simulink model "sun_vector_test_vallado"  (R2016b)
settings: Solver=VariableStepAuto  StartTime=0.0  StopTime=1  RelTol=1e-3
values from neighbouring files (symbols this model uses):
  JD_cent = (JD - J2000)/36525    (= -0.0487748117728)    [sun_vector_test_init.m]
  r_eci = [ 0; -4464.696; -5102.509 ] * 1e3    [sun_vector_test_init.m]
undefined symbols (not defined in the file or in its folder): sun_vector_lib
settings Model: Creator=taylorreynolds  LastModifiedBy=taylorreynolds

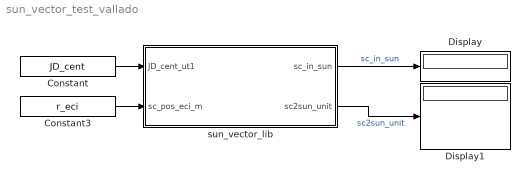
== system sun_vector_test_vallado ==
  Constant : Constant  Value=JD_cent
  Constant3 : Constant  Value=r_eci
  Display : Display
  Display1 : Display
  sun_vector_lib : Subsystem  AncestorBlock=sun_vector_lib/sun_vector_lib
  wires:
  Constant/1 -> sun_vector_lib/1(JD_cent_ut1)
  sun_vector_lib/1(sc_in_sun) -> Display/1  "sc_in_sun"
  sun_vector_lib/2(sc2sun_unit) -> Display1/1  "sc2sun_unit"
  Constant3/1 -> sun_vector_lib/2(sc_pos_eci_m)

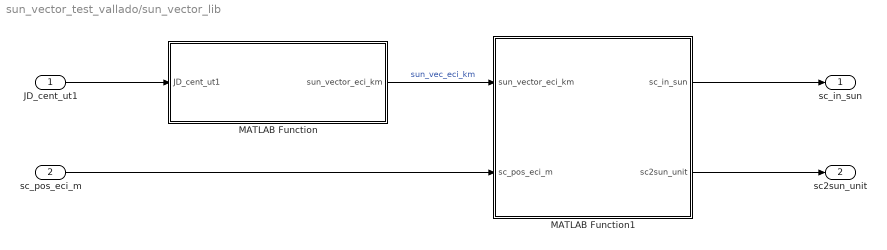
== system sun_vector_test_vallado/sun_vector_lib ==
  JD_cent_ut1 : Inport
  sc_pos_eci_m : Inport  Port=2
  MATLAB Function : MATLAB Function  TreatAsAtomicUnit=on
  MATLAB Function1 : MATLAB Function  TreatAsAtomicUnit=on
  sc_in_sun : Outport
  sc2sun_unit : Outport  Port=2
  wires:
  MATLAB Function1/1(sc_in_sun) -> sc_in_sun/1
  MATLAB Function1/2(sc2sun_unit) -> sc2sun_unit/1
  sc_pos_eci_m/1 -> MATLAB Function1/2(sc_pos_eci_m)
  MATLAB Function/1(sun_vector_eci_km) -> MATLAB Function1/1(sun_vector_eci_km)  "sun_vec_eci_km"
  JD_cent_ut1/1 -> MATLAB Function/1(JD_cent_ut1)

== matlab function sun_vector_test_vallado/sun_vector_lib/MATLAB Function ==
  data: JD_cent_ut1 input; sun_vector_eci_km output
function sun_vector_eci_km = sun_vector(JD_cent_ut1)
% ----------------------------------------------------------------------- %
% UW HuskySat-1, ADCS Team
% Algorithm to find the sun vector in the ECI frame. Based on algorithm 29 
%   from Vallado 4e (pp. 279-280).
%
% T. Reynolds -- 2.23.18
% ----------------------------------------------------------------------- %

% Constants
AU2KM   = 149597870.700; 
DEG2RAD     = pi/180.0;
TWOPI   = 2*pi;

% Mean longitude in a mean-equator of date frame
mean_long_sun  = rem(280.460 + 36000.771*JD_cent_ut1,360); % [deg]

% Mean anomaly for the sun. Low precision formula since we're approximating
% T_TDB with T_UT1.
mean_anom_sun       = rem(357.5291092 + 35999.05034*JD_cent_ut1,360); %[deg]
mean_anom_sun_rad   = mod(DEG2RAD*mean_anom_sun,TWOPI);

% Approximate the ecliptic longitude of the sun
long_eclp       = mean_long_sun + 1.914666471*sin(mean_anom_sun_rad) + ...
                    0.019994643*sin(2*mean_anom_sun_rad); %[deg]
long_eclp       = rem(long_eclp,360); % [rad]   
long_eclp_rad   = mod(DEG2RAD*long_eclp,TWOPI);
       
% Assume the ecliptic latitude is zero
lat_eclp     = 0; %[deg]

% Approximate the obliquity of the ecliptic using
oblq        = 23.439291 - 0.0130042*JD_cent_ut1;
oblq_rad    = DEG2RAD*oblq;

% Find the distance in AU from E to S
r           =  1.000140612 - 0.016708617*cos(mean_anom_sun_rad) - ...
                    0.000139589*cos(2*mean_anom_sun_rad);
x_MOD_km    = r*cos(long_eclp_rad)*AU2KM;
y_MOD_km    = r*cos(oblq_rad)*sin(long_eclp_rad)*AU2KM;
z_MOD_km    = r*sin(oblq_rad)*sin(long_eclp_rad)*AU2KM;

sun_vector_mod_km = [x_MOD_km; y_MOD_km; z_MOD_km];

% Convert to ECI (mean-equator-mean-equinox) frame 
sun_vector_eci_km   = mod2eci(sun_vector_mod_km,JD_cent_ut1);

end

function vec_eci = mod2eci(vec_mod,JD_cent_ut1)

[prec,~,~,~,~] = precess ( JD_cent_ut1 );

vec_eci = prec*vec_mod;

end

function [prec,psia,wa,ea,xa] = precess ( ttt )
% " to rad
convrt = pi / (180.0*3600.0);

% ------------------ iau 03 precession angles -------------------
oblo =  84381.406; % "
psia =  (((( -0.0000000951 * ttt + 0.000132851 ) * ttt - 0.00114045 ) *...
                        ttt - 1.0790069 ) * ttt + 5038.481507 ) * ttt; % "
wa   =  ((((  0.0000003337 * ttt - 0.000000467 ) * ttt - 0.00772503 ) *...
                        ttt + 0.0512623 ) * ttt -    0.025754 ) * ttt + oblo;
ea   =  (((( -0.0000000434 * ttt - 0.000000576 ) * ttt + 0.00200340 ) *...
                        ttt - 0.0001831 ) * ttt -   46.836769 ) * ttt + oblo;
xa   =  (((( - 0.0000000560 * ttt + 0.000170663 ) * ttt - 0.00121197 ) *...
                        ttt - 2.3814292 ) * ttt +   10.556403 ) * ttt;

zeta =  (((( - 0.0000003173 * ttt - 0.000005971 ) * ttt + 0.01801828 ) *...
                ttt + 0.2988499 ) * ttt + 2306.083227 ) * ttt + 2.650545; % "
theta=  (((( - 0.0000001274 * ttt - 0.000007089 ) * ttt - 0.04182264 ) *...
                ttt - 0.4294934 ) * ttt + 2004.191903 ) * ttt;
z    =  ((((   0.0000002904 * ttt - 0.000028596 ) * ttt + 0.01826837 ) *...
                ttt + 1.0927348 ) * ttt + 2306.077181 ) * ttt - 2.650545;

% convert all units to rad
psia = psia  * convrt; % rad
wa   = wa    * convrt;
ea   = ea    * convrt;
xa   = xa    * convrt;

oblo = oblo * convrt; % " to rad
a4  = rot3mat(-xa);
a5  = rot1mat(wa);
a6  = rot3mat(psia);
a7  = rot1mat(-oblo);
prec = a7*a6*a5*a4;

end % precess

function DCMx = rot1mat(x_rad)

s   = sin( x_rad );
c   = cos( x_rad );

DCMx    = [ 1   0   0
            0   c   s;
            0  -s   c ];

end

function DCMz   = rot3mat(z_rad)

s   = sin( z_rad );
c   = cos( z_rad );

DCMz    = [ c   s   0;
           -s   c   0;
            0   0   1 ];

end

== matlab function sun_vector_test_vallado/sun_vector_lib/MATLAB Function1 ==
  data: sun_vector_eci_km input; sc_in_sun output; sc2sun_unit output; sc_pos_eci_m input
function [sc_in_sun,sc2sun_unit] = sc_in_sun(sun_vector_eci_km,sc_pos_eci_m)
% ----------------------------------------------------------------------- %
% UW HuskySat-1, ADCS Team
%
% Function to find both the vector from the s/c to the sun, and determine
% if we are in eclipse or not. Based on algorithm 35 from Vallado 4e, pp
% 308.
%
% T. Reynolds -- 2.23.18
% ----------------------------------------------------------------------- %

% Constants
M2KM        = 1e-3;
ECCE2       = 0.006694385000;
RE          = 6378.137; % km
TRUE        = 1;
FALSE       = 0;
LOS         = FALSE;
% -----

% Convert both inputs to km
r1  = sc_pos_eci_m*M2KM;
r2  = sun_vector_eci_km;
magr1   = mag(r1);
magr2   = mag(r2);

% Main Function
% For ellipsoidal earth
temp    = 1.0 / sqrt(1.0 - ECCE2);
r1(3)   = r1(3) * temp;
r2(3)   = r2(3) * temp;

asqrd   = magr1 * magr1;
bsqrd   = magr2 * magr2;
adotb   = dot( r1,r2 );

if( abs(asqrd + bsqrd - 2.0*adotb) < 0.0001 )
    tmin = 0.0;
else
    tmin = (asqrd - adotb) / (asqrd + bsqrd - 2.0*adotb);
end

if( (tmin < 0.0) || (tmin > 1.0) )
    LOS = TRUE;
else
    dist2   = ( (1.0-tmin)*asqrd + adotb*tmin )/RE^2;
    if( dist2 > 1.0 )
        LOS = TRUE;
    else
        LOS = FALSE;
    end
end

sc2sun_unit     = (r2-r1)/norm(r2-r1);
sc_in_sun       = LOS;
end

function mag = mag( vec )
    temp = vec(1)*vec(1) + vec(2)*vec(2) + vec(3)*vec(3);
    if( abs( temp ) >= 1e-16 )
        mag = sqrt( temp );
    else
        mag = 0.0;
    end
end
